simulink model "DiversCODAGES1"  (R2020a)
settings: Solver=FixedStepDiscrete  StartTime=0.0  StopTime=inf  RelTol=1e-3
libraries: commrandsrc2 x1, commutil2 x1
settings Model: Creator=Vincent  LastModifiedBy=J-MENTION
settings DataIOCC: LimitDataPoints=on  SaveFormat=Array  SignalLoggingSaveFormat=ModelDataLogs  SaveOutput=off  SignalLogging=off  SaveTime=off  ReturnWorkspaceOutputs=off
settings OptimizationCC: ExpressionDepthLimit=2147483647  InitFltsAndDblsToZero=on  LifeSpan=inf
settings DebuggingCC: AlgebraicLoopMsg=error  UnderspecifiedInitializationDetection=Classic  MergeDetectMultiDrivingBlocksExec=none  SolverPrmCheckMsg=warning  FcnCallInpInsideContextMsg=warning  StateNameClashWarn=warning  SFUnexpectedBacktrackingDiag=warning  SFNoUnconditionalDefaultTransitionDiag=warning  SFExecutionAtInitializationDiag=none  ArithmeticOperatorsInVariantConditions=warning
settings HardwareCC: ProdBitPerPointer=32  ProdBitPerSizeT=32  ProdBitPerPtrDiffT=32  ProdLargestAtomicFloat=None  ProdIntDivRoundTo=Undefined  ProdEndianess=Unspecified  ProdWordSize=32  ProdHWDeviceType=32-bit Generic
settings ModelReferenceCC: PropagateSignalLabelsOutOfModel=off
settings SFSimCC: SimUseLocalCustomCode=off  CustomCodeUndefinedFunction=UseInterfaceOnly
settings RTWCC: RTWUseLocalCustomCode=off
settings CodeAppCC: StateflowObjectComments=on
settings GRTTargetCC: TargetLangStandard=C89/C90 (ANSI)  CombineOutputUpdateFcns=off  GRTInterface=on
settings ConfigComp: CovMetricSettings=dw  CovHtmlReporting=on  CovSaveCumulativeToWorkspaceVar=on  CovSaveSingleToWorkspaceVar=on  CovExternalEMLEnable=off

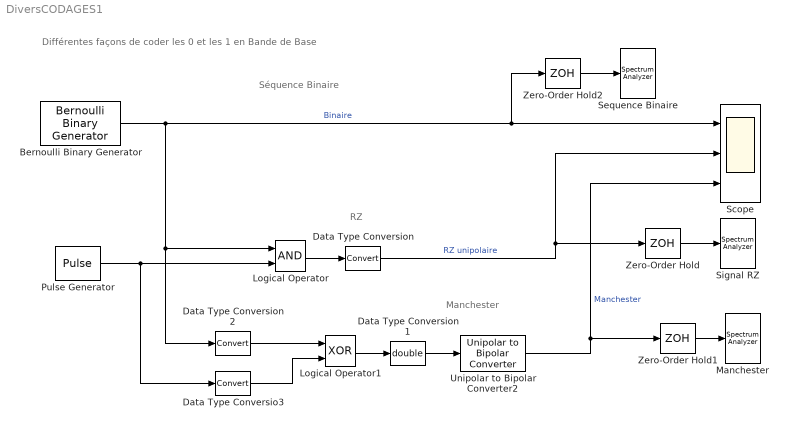
== system DiversCODAGES1 ==
  note: Différentes façons de coder les 0 et les 1 en Bande de Base
  note: Séquence Binaire
  note: RZ
  note: Manchester
  Bernoulli Binary Generator : commrandsrc2/Bernoulli Binary Generator  P=0.5  seed=61  Ts=1e-3  frameBased=off  sampPerFrame=1  orient=off  outDataType=double
      settings: SourceProductBaseCode=CM
  Data Type Conversio3 : DataTypeConversion
  Data Type Conversion : DataTypeConversion
  Data Type Conversion1 : DataTypeConversion  OutDataTypeStr=double
  Data Type Conversion2 : DataTypeConversion
  Logical Operator : Logic  AllPortsSameDT=off  OutDataTypeStr=boolean
  Logical Operator1 : Logic  Operator=XOR
  "Manchester " : SpectrumAnalyzer
  Pulse Generator : DiscretePulseGenerator  SampleTime=500e-6
  Scope : Scope  NumInputPorts=3
  "Sequence Binaire " : SpectrumAnalyzer
  "Signal RZ " : SpectrumAnalyzer
  Unipolar to Bipolar Converter2 : commutil2/Unipolar to Bipolar Converter  M=2  polarity=Positive  dataType=Same as input
  Zero-Order Hold : ZeroOrderHold  SampleTime=1e-4
  Zero-Order Hold1 : ZeroOrderHold  SampleTime=1e-4
  Zero-Order Hold2 : ZeroOrderHold  SampleTime=1e-4
  wires:
  Bernoulli Binary Generator/1 -> Logical Operator/1, Data Type Conversion2/1, Zero-Order Hold2/1, Scope/1  "Binaire"
  Pulse Generator/1 -> Logical Operator/2, Data Type Conversio3/1
  Logical Operator/1 -> Data Type Conversion/1
  Data Type Conversion1/1 -> Unipolar to Bipolar Converter2/1
  Logical Operator1/1 -> Data Type Conversion1/1
  Data Type Conversion2/1 -> Logical Operator1/1
  Data Type Conversio3/1 -> Logical Operator1/2
  Zero-Order Hold/1 -> "Signal RZ "/1
  Zero-Order Hold1/1 -> "Manchester "/1
  Data Type Conversion/1 -> Scope/2, Zero-Order Hold/1  "RZ unipolaire"
  Unipolar to Bipolar Converter2/1 -> Zero-Order Hold1/1, Scope/3  "Manchester"
  Zero-Order Hold2/1 -> "Sequence Binaire "/1
